simulink model "sm_stewart_platform"  (R2019a)
settings: Solver=ode45  StartTime=0.0  StopTime=40  MaxStep=0.001  RelTol=1e-3  EnableMultiTasking=on
model workspace (MAT data in the model file):
  g_density = 5
undefined symbols (not defined in the file or in its folder): B, nom_length, P, X, Y, Z
libraries: sm_lib x20, sm_stewart_platform_lib x8, nesl_utility x4
(part 1 of 3)
Description:
  | Stewart Platform
  | 
  | This model shows a Stewart platform manipulator that can track a
  | parameterized reference trajectory. The shape, size, and kinematics of
  | the manipulator are highly configurable.
  | 
  | The reference trajectory is
  | specified in 6-D pose space, and an inverse kinematics module
  | converts it into one through 6-D leg position space.  A generic PID
  | controller attempts to drive the manipulator along the desired
  | trajectory.
  | 
  | 
  | Copyright 2011-2018 The MathWorks, Inc.
settings Model: FPTRunName=Active  Creator=MathWorks  LastModifiedBy=Cybaster
settings DataIOCC: LimitDataPoints=on  SaveFormat=Array  SignalLoggingSaveFormat=ModelDataLogs  ReturnWorkspaceOutputs=off
settings OptimizationCC: ExpressionDepthLimit=2147483647  LifeSpan=inf
settings DebuggingCC: UnderspecifiedInitializationDetection=Classic  MergeDetectMultiDrivingBlocksExec=none  SolverPrmCheckMsg=warning  FcnCallInpInsideContextMsg=warning  StateNameClashWarn=warning  SFUnexpectedBacktrackingDiag=warning  SFNoUnconditionalDefaultTransitionDiag=warning  SFExecutionAtInitializationDiag=none  ArithmeticOperatorsInVariantConditions=warning
settings HardwareCC: ProdBitPerPointer=32  ProdBitPerSizeT=32  ProdBitPerPtrDiffT=32  ProdLargestAtomicFloat=None  ProdIntDivRoundTo=Undefined  ProdEndianess=Unspecified  ProdWordSize=32  ProdHWDeviceType=32-bit Generic
settings ModelReferenceCC: PropagateSignalLabelsOutOfModel=off
settings SFSimCC: SimUseLocalCustomCode=off
settings RTWCC: RTWUseLocalCustomCode=off
settings CodeAppCC: StateflowObjectComments=on
settings GRTTargetCC: TargetLangStandard=C89/C90 (ANSI)  GeneratePreprocessorConditionals=Disable all  CombineOutputUpdateFcns=off  GRTInterface=on
settings ConfigComp: CovMetricSettings=dw  CovHtmlReporting=on  CovSaveCumulativeToWorkspaceVar=on  CovSaveSingleToWorkspaceVar=on  CovExternalEMLEnable=off
settings SimscapeCC: SimscapeNormalizeSystem=off  SimscapeLogDataHistory=15000
settings ConfigurationSet: Description=SimMechanics 2G

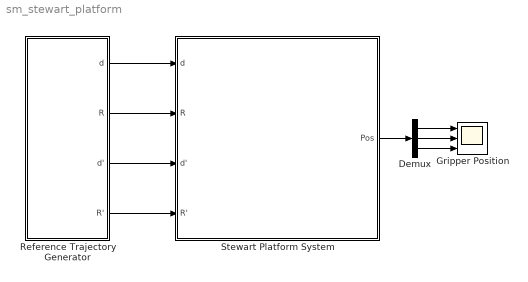
== system sm_stewart_platform ==
  Demux : Demux  Outputs=3
  Gripper Position : Scope  NumInputPorts=3
  Reference Trajectory Generator : Subsystem  mask(3-D Transform Trajectory Generator){Ax=0, wx=0, px=0, kx=0, Ay=0, wy=0, py=0, ky=0, Az=4, wz=180 / 10, pz=-90, kz=75, Aa=10, wa=360 * 3 / 10, pa=0, ka=0, Ab=10, wb=360 * 3 / 10, pb=-90, kb=0, Ac=0, wc=0, pc=0, kc=0}
      mask prompts: Ax "X Displacement Amplitude (cm)"; wx "X Displacement Frequency (deg / s)"; px "X Displacement Phase (deg)"; kx "X Displacement Offset (cm)"; Ay "Y Displacement Amplitude (cm)"; wy "Y Displacement Frequency (deg / s)"; py "Y Displacement Phase (deg)"; ky "Y Displacement Offset (cm)"; Az "Z Displacement Amplitude (cm)"; wz "Z Displacement Frequency (deg / s)"; pz "Z Displacement Phase (deg)"; kz "Z Displacement Offset (cm)"; Aa "X Rotation Amplitude (deg)"; wa "X Rotation Frequency (deg / s)"; pa "X Rotation Phase (deg)"; ka "X Rotation Offset (deg)"; Ab "Y Rotation Amplitude (deg)"; wb "Y Rotation Frequency (deg / s)"; pb "Y Rotation Phase (deg)"; kb "Y Rotation Offset (deg)"; Ac "Z Rotation Amplitude (deg)"; wc "Z Rotation Frequency (deg / s)"; pc "Z Rotation Phase (deg)"; kc "Z Rotation Offset (deg)"
      mask help: Tool for generating a wide variety of trajectories for a time-varying, 3-D rigid transformation between two frames.
      mask Help:
      | A <em>3-D Transform Trajectory Generator</em> is a tool for generating a wide variety of trajectories for a time-varying, 3-D rigid transformation between two frames.
      | 
      | A rigid transformation between two frames is characterized by a displacement vector and a rotation matrix.  Each of these can be parameterized with three scalar coordinates.  This block allows these six scalar coordinates to be parametrically specified as arbitrary sinusoidal functions of time.  The resulting displacement vector and rotation matrix, and their first derivatives are provided on the output ports.
      | 
      | <h3>Sinsoidal Functions</h3>
      | 
      | An arbitrary sinusoidal function of time is given by
      | 
      |     f(t) = A sin (w t + p) + k,
      | 
      | where <em>t</em> is time, and <em>A, w, p,</em> and <em>k</em> are scalar constants with the following meanings:
      | <ul>
      | <li> <em>A</em> is the <em>amplitude</em> of the sinusoid.
      | <li> <em>w</em> is the <em>angular frequency</em> of the sinusoid.
      | <li> <em>p</em> is the <em>phase</em> of the sinusoid.
      | <li> <em>k</em> is the <em>offset</em> of the sinusoid.
      | </ul>
      | 
      | <h3>Rigid Transformations</h3>
      | 
      | The time-varying, 3-D rigid transformation provided on the output ports of this block is, in turn, a function of scalar functions.  The displacement vector of the rigid transformation is given by:
      | 
      |     <b>d</b>(t) = [ x(t), y(t), z(t) ]^T
      | 
      | where x(t), y(t), and z(t) are scalar functions of time.
      | 
      | The rotation matrix of the rigid transformation is given by:
      | 
      |     <b>R</b>(t) = <b>R_x</b>(a(t)) <b>R_y</b>(b(t)) <b>R_z</b>(c(t)),
      | 
      | where a(t), b(t), and c(t) are scalar functions of time, and <b>R_x</b>, <b>R_y</b>, and <b>R_z</b> are rotations about the x, y, and z axes, respectively.
      | 
      | Note that this is an Euler angle parameterization of rotation.  The final rotation maps directions from a rotating frame F to a fixed frame G.  Beginning with F and G in an aligned configuration, the full rotation can be realized as a sequence of three rotations: first rotate F about its x-axis, then rotate F about its y-axis, and finally rotate F about its z-axis.  Alternatively, the rotation can be realized in a fixed-frame manner: first rotate F about G's z-axis, then rotate F about G's y-axis, and finally rotate F about G's z-axis. Both interpretations are correct.
      | 
      | The six scalar functions x(t), y(t), z(t), a(t), b(t), and c(t) are all arbitrary sinusoidal functions.  Each is parameterized by the four constants described in the preceding section.  This block computes these functions, and uses them to build the displacement vector, the rotation matrix, and the first time derivatives of these quantities.
      | 
      | 
      | <h3>Parameters</h3>
      | 
      | Each of the six parameter tabs defines four scalar parameters that together specify an arbitrary sinusoidal function of time, as described above.  The six tabs are:
      | 
      | <ul>
      | 
      | <li> <b>dx</b> Specifies the x-component of the displacement vector as a sinusoidal function of time.
      | 
      | <li> <b>dy</b> Specifies the y-component of the displacement vector as a sinusoidal function of time.
      | 
      | <li> <b>dz</b> Specifies the z-component of the displacement vector as a sinusoidal function of time.
      | 
      | <li> <b>Rx</b> Specifies the scalar rotation about the x-axis, part of the three-stage rotation sequence, as a sinusoidal function of time.
      | 
      | <li> <b>Ry</b> Specifies the scalar rotation about the y-axis, part of the three-stage rotation sequence, as a sinusoidal function of time.
      | 
      | <li> <b>Rz</b> Specifies the scalar rotation about the z-axis, part of the three-stage rotation sequence, as a sinusoidal function of time.
      | 
      | </ul>
      | 
      | <h3>Ports</h3>
      | 
      | <ul>
      | 
      | 
      | <li><b>d</b> The displacement vector of the time-varying, 3-D rigid transformation as a signal output.  This value is a 3 x 1 vector in units of centimeters.
      | 
      | <li><b>R</b> The rotation matrix of the time-varying, 3-D rigid transformation as a signal output.  This value is a 3 x 3 orthogonal matrix with +1 determinant.
      | 
      | <li><b>d'</b> The first time derivative of the signal appearing on the <em>d</em> port: a 3 x 1 vector in units of centimeters/second.
      | 
      | <li><b>R'</b> The first time derivative of the signal appearing on the <em>R</em> port: a 3 x 3 matrix.
      | 
      | </ul>
  Stewart Platform System : Subsystem  mask(Stewart Platform System){base_rad=28, base_thick=8, platform_rad=18, platform_thick=2, hex_skew=-0.25, upper_leg_len=10, lower_leg_len=14, leg_rad=3, collar_thick=0.5, gripper_height=30, claw_length=8, claw_width=3, claw_thick=1, end_eff_base_thick=2, flange_len=3, flange_width=2.25, flange_thick=.8, ic_R=eye(3), ic_d=[0 0 71]', Kp=300, Ki=20, Kd=5}
      mask prompts: base_rad "Base Radius  (cm)"; base_thick "Base Thickness (cm)"; platform_rad "Platform Radius (cm)"; platform_thick "Platform Thickness (cm)"; hex_skew "Hexagon Skew"; upper_leg_len "Upper Leg Length (cm)"; lower_leg_len "Lower Leg Length (cm)"; leg_rad "Leg Radius (cm)"; collar_thick "Collar Thickness (cm)"; gripper_height "Gripper Height (cm)"; claw_length "Claw Length (cm)"; claw_width "Claw Width (cm)"; claw_thick "Claw Thickness (cm)"; end_eff_base_thick "Base Thickness (cm)"; flange_len "Flange Length (cm)"; flange_width "Flange Width (cm)"; flange_thick "Flange Thickness (cm)"; ic_R "Rotation Matrix [3 x 3]"; ic_d "Displacement Vector (cm) [3 x 1]"; Kp "Controller Proportional Gain (N / cm)"; Ki "Controller Integral Gain (N / (cm s))"; Kd "Controller Derivative Gain (N / (cm / s)))"
      mask help:
      | Models a complete Stewart platform manipulator system.  The system can be driven to position and orient a special gripper frame according to specified trajectories.
      |
      | The system comprises a mechanical manipulator, an inverse kinematics module, and a control system.
      mask init:
      | params = struct( ...
      |     'base_thick',        base_thick,     ...
      |     'base_radius',       base_rad,       ...
      |     'platform_thick',    platform_thick, ...
      |     'platform_radius',   platform_rad,   ...
      |     'skew',              hex_skew,       ...
      |     'flange_length',     flange_len,     ...
      |     'flange_width',      flange_width,   ...
      |     'flange_thick',      flange_thick,   ...
      |     'leg_radius',        leg_rad,        ...
      |     'upper_leg_length',  upper_leg_len,  ...
      |     'lower_leg_length',  lower_leg_len,  ...
      |     'gripper_height',    gripper_height  ...
      |     );
      | 
      | [B, P, nom_length] = sm_stewart_platform_setup(params);
      | 
      | lengths = sm_stewart_platform_ik(B, P, nom_length, ic_R, ic_d);
      mask Help:
      | A <em>Stewart Platform System</em> models a complete Stewart platform manipulator system.  The system can be driven to position and orient a special gripper frame according to specified trajectories.
      | 
      | <h3>Subsystems</h3>
      | 
      | A Stewart platform system comprises three primary subsystems:
      | 
      | <ol>
      | 
      | <li><b>Manipulator</b> The manipulator is the Simscape Multibody subsystem describing the mechanical structure of the Stewart platform.  The manipulator contains two hexagonal plates, a lower base plate and an upper platform plate, connected by six articulated legs.  The base plate is anchored to the world frame, and the platform plate is controlled to position and orient the gripper frame. The manipulator component provides sensing and actuation signals to interface to a controller.
      | 
      |   The manipulator is highly parameterized.  Most parameters of the Stewart platform system are physical lengths and other parameters that control the shapes and sizes of the components of the manipulator. By varying these parameters, a wide range of Stewart platform manipulators can be realized.
      | 
      | <li><b>Inverse Kinematics (IK) Module</b> The inverse kinematics module is a pure Simulink subsystem that maps time-varying signals describing the desired position and orientation of the gripper frame into time-varying scalar signals specifying the positions and velocities of the prismatic primitives of the leg joints.  This is an essential component of a complete Stewart platform system because the user of the system typically expresses a desired trajectory in the 6-D space of positions and orientations of the gripper frame, but the manipulator control is simplest in the 6-D space of leg joint positions. The IK module forms the bridge between these two spaces.
      | 
      |   The mathematics performed within the IK module is heavily dependent on the physical parameters that determine the shape and size of the manipulator itself.  Most of the parameters that govern the manipulator are also used within the IK module.
      | 
      | <li><b>Control System</b> The control system is a pure Simulink subsystem that attempts to drive the gripper frame along its desired trajectory by controlling the positions of the prismatic primitives of the leg joints. It uses a standard PID control scheme, with gains specified by Stewart platform system parameters.  The control uses no information about the forward or inverse kinematics of the platform; it simply tries to drive a point along a trajectory in 6-D space.
      | 
      |   The controller takes both the desired and actual leg position vectors and the first derivatives of these quantities.  It generates a 6-D commanded force output that can be used to drive the six leg lengths to thei desired values.
      | 
      |   Because the size and shape of the Stewart platform manipulator can vary significantly depending on the parameter settings, the controller gains may need to be adjusted in order to control the manipulator to the desired trajectory.
      | 
      | </ol>
      | 
      | <h3>Base and Platform Plates</h3>
      | 
      | The <em>Plates</em> tab parameters specify the geometry of the base and platform hexagon plates of the Stewart platform manipulator.  See the documentation of the <em>Hexagon Plate</em> library block for details.
      | 
      | <ul>
      | 
      | <li> <b>Base Radius</b> The radius of the base plate.  The vertices of the hexagonal cross section all lie on a circle of this radius.
      | 
      | <li> <b>Base Thickness</b> The thickness of the base plate.
      | 
      | <li> <b>Platform Radius</b> The radius of the platform plate.  The vertices of the hexagonal cross section all lie on a circle of this radius.
      | 
      | <li> <b>Platform Thickness</b> The thickness of the platform plate.
      | 
      | <li> <b>Hexagon Skew</b> The common skew factor of the base and platform plates. This value, in the range (-0.5, +0.5), determines the shape of the three-fold symmetric hexagons.  A zero skew factor produces regular hexagons.  As the skew factor magnitude increases, the hexagons become more triangular.
      | 
      | </ul>
      | 
      | <h3>Legs</h3>
      | 
      | The <em>Legs</em> tab parameters specify the common geometry of the six legs of the Stewart platform manipulator.  See the documentation of the <em>Leg</em> library block for details.
      | 
      | <ul>
      | 
      | <li> <b>Upper Leg Length</b> The length of the upper leg, including its end collars.
      | 
      | <li> <b>Lower Leg Length</b> The length of the lower leg, including its end collars.
      | 
      | <li> <b>Leg Radius</b> The common radius of the upper and lower leg segments. Each segment's cross section is a regular hexagon inscribed in a circle of this radius.
      | 
      | <li> <b>Collar Thickness</b> The thickness of the hexagonal collars adjoined to the ends of each leg segment.
      | 
      | </ul>
      | 
      | <h3>End Effector</h3>
      | 
      | The <em>End Eff</em> tab parameters specify the geometry of the end effector attached to the platform plate of the Stewart platform manipulator. See the documentation of the <em>End Effector</em> block within the <em>Manipulator</em> subsystem for details.
      | 
      | <ul>
      | 
      | <li> <b>Gripper Height</b> The vertical distance from the origin of the gripper frame to the top surface of the movable platform plate.
      | 
      | <li> <b>Claw Length</b> The length (height) of the trapezoidal claws of the gripper.
      | 
      | <li> <b>Claw Width</b> The width of the trapezoidal claws of the gripper where they attach to the gripper base.
      | 
      | <li> <b>Claw Thickness</b> The thickness of the trapezoidal claws of the gripper.
      | 
      | <li> <b>Base Thickness</b> The thickness of the triangular gripper base.
      | 
      | </ul>
      | 
      | <h3>Flanges</h3>
      | 
      | The <em>Flanges</em> tab parameters specify the common geometry of the 48 flanges attached to the hexagonal plates and legs of the Stewart platform manipulator.  Each of the 12 universal joints is supported by four flanges.  See the documentation of the <em>Flange</em> library block for details.
      | 
      | <ul>
      | 
      | <li> <b>Flange Length</b> The length of the rectangular prism portion of the flanges.
      | 
      | <li> <b>Flange Width</b> The width of the rectangular prism portion of the flanges.
      | 
      | <li> <b>Flange Thickness</b> The thickness of the flanges.
      | 
      | </ul>
      | 
      | <h3>Initial Conditions</h3>
      | 
      | The <em>IC</em> tab parameters specify the initial conditions of the Stewart Platform manipulator for simulation.  Specifically, these specify the <em>position</em> of the manipulator; the simulation always starts from a rest (zero velocity) state.
      | 
      | The initial position is defined by specifying pose of the gripper frame relative to the world frame.  This is typically a convenient parameterization for a user of the manipulator.  The world frame is also the reference frame of the manipulator base plate.  This is a frame with origin at the center of the manipulator base (which is in its interior), and with z-axis pointed directly upward.
      | 
      | An Update Diagram (Ctrl-D) operation will attempt to assemble the manipulator in the specified initial position.  Some initial positions may be incompatible with the kinematics of the manipulator, based on other parameter settings.  In such cases, the assembly will fail.
      | 
      | Also note that if the initial position differs significantly from the desired trajectory (specified through the input signal ports) at time zero, the manipulator's motion may be subject to large transients at the start of simulation.
      | 
      | <ul>
      | 
      | <li> <b>Rotation Matrix</b> The rotation matrix mapping directions in the gripper frame to directions in the world frame.  This should be a 3 x 3 orthogonal matrix determinant +1.  The columns of this matrix are the canonical i, j, and k unit vectors of the gripper frame resolved in world frame coordinates.
      | 
      | <li> <b>Displacement Vector</b> The location of the origin of the gripper frame in world frame coordinates.  This should be a 3 x 1 column vector.  The z-coordinate should generally be positive, on the order of the nominal lengths of the legs.
      | 
      | </ul>
      | 
      | If the rotation matrix is the identity and the x- and y-coordinates of the displacement vector are zero, the initial configuration of the manipulator will be symmetric with all leg positions equal.
      | 
      | <h3>Controller Gains</h3>
      | 
      | The <em>Control</em> tab parameters specify the gains of the internal controller used to control the manipulator's pose according to a specified trajectory.  The controller uses a generic PID control scheme.  The gains may need to be adjusted to be appropriate if the parameters governing the size and kinematics of the manipulator are changed significantly.
      | 
      | See the documentation of the <em>Controller</em> subsystem for details.
      | 
      | <ul>
      | 
      | <li> <b>Controller Proportional Gain</b> The proportional (P) gain of the internal PID controller.
      | 
      | <li> <b>Controller Integral Gain</b> The integral (I) gain of the internal PID controller.
      | 
      | <li> <b>Controller Derivative Gain</b> The derivative (D) gain of the internal PID controller.
      | 
      | </ul>
      | 
      | 
      | 
      | <h3>Ports</h3>
      | 
      | <ul>
      | 
      | <li><b>d</b> The desired displacement vector of the gripper frame relative to the world frame as a signal input.  This value should be a 3 x 1 vector in units of centimeters.  It specifies the desired origin of the gripper frame in world frame coordinates as a function of time.  This signal is analogous to the <em>Displacement Vector</em> on the <em>IC</em> parameter tab.
      | 
      | <li><b>R</b> The desired rotation matrix from the gripper frame to the world frame as a signal input.  This value should be a 3 x 3 orthogonal matrix with +1 determinant.  The columns of this matrix are the canonical i, j, and k unit vectors of the gripper frame resolved in world frame coordinates, specified as functions of time.  This signal is analogous to the <em>Rotation Matrix</em> on the <em>IC</em> parameter tab.
      | 
      | <li><b>d'</b> The first time derivative of the desired displacement vector of the gripper frame relative to the world frame as a signal input.  This value should be the first time derivative of the signal provided on the <em>d</em> port: a 3 x 1 vector in units of centimeters/second. It specifies the velocity of the origin of the gripper frame in  world frame coordinates as a function of time.
      | 
      | <li><b>R'</b> The first time derivative of the desired rotation matrix from the gripper frame to the world frame as a signal input.  This value should be the first time derivative of the signal provided on the <em>R</em> port: a 3 x 3 matrix.
      | 
      | <li><b>Pos</b> The position of the gripper with respect to the world frame as a 3 x 1 position vector in units of centimeters.
      | </ul>
      | 
      | <!--  LocalWords:  Eff IC Ctrl IK
      |  -->
      mask Display:
      | image(imread('sm_stewart_platform_system.png'))
      | color('yellow')
      | port_label('Input', 1, 'd')
      | port_label('Input', 2, 'R')
      | port_label('Input', 3, 'd''')
      | port_label('Input', 4, 'R''')
      | port_label('Output', 1, 'Pos')
  wires:
  Reference Trajectory Generator/1(d) -> Stewart Platform System/1(d)
  Reference Trajectory Generator/2(R) -> Stewart Platform System/2(R)
  Reference Trajectory Generator/3(d') -> Stewart Platform System/3(d')
  Reference Trajectory Generator/4(R') -> Stewart Platform System/4(R')
  Stewart Platform System/1(Pos) -> Demux/1
  Demux/1 -> Gripper Position/1
  Demux/2 -> Gripper Position/2
  Demux/3 -> Gripper Position/3

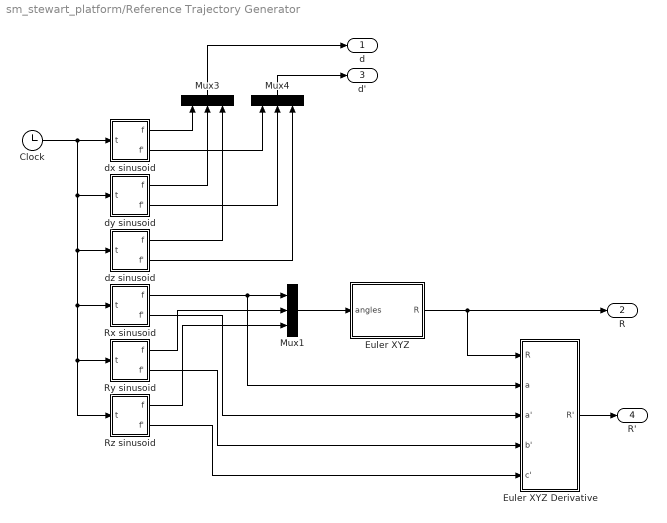
== system sm_stewart_platform/Reference Trajectory Generator ==
  Clock : Clock
  Euler XYZ : Subsystem  mask(Euler XYZ){}
      mask help: Converts a set of Euler angles to the corresponding rotation matrix from rotated frame to fixed frame coordinates.
      mask Help:
      | An <em>Euler XYZ</em>  block converts a set of Euler angles to the corresponding
      |   rotation matrix from rotated frame to fixed frame coordinates.
      | 
      | Arbitrary 3-D rotations can be parameterized by a vector of three Euler angles:
      |   a, b, and c.  The resulting rotation is given by
      | 
      |     <b>R</b> = <b>R_x</b>(a) <b>R_y</b>(b) <b>R_z</b>(c).
      | 
      | where <b>R_x</b>, <b>R_y</b>, and <b>R_z</b> are rotations about the x, y, and z
      | axes, respectively.
      | 
      | The complete rotation <b>R</b> maps directions from a rotated frame F to a
      | fixed frame G.  Beginning with F and G in an aligned configuration, the full
      | rotation can be realized as a sequence of three rotations: first rotate F
      | about its x-axis, then rotate F about its y-axis, and finally rotate F about its
      | z-axis.  Alternatively, the rotation can be realized in a fixed-frame manner:
      | first rotate F about G's z-axis, then rotate F about G's y-axis, and finally
      | rotate F about G's z-axis.  Both interpretations are correct.
      | 
      | 
      | <h3>Ports</h3>
      | 
      | <ul>
      | 
      | <li> <b>angles</b> The Euler angles a, b, and c (in that order) as a 3-vector
      |   with units of radians.
      | 
      | <li> <b>R</b> The resulting rotation matrix.  This matrix is always a 3 x 3
      | orthogonal matrix with a +1 determinant.
      | 
      | </ul>
  Euler XYZ Derivative : Subsystem  mask(Euler XYZ Derivative){}
      mask help: Computes the first time derivative of a rotation matrix specified by a set of Euler angles.
      mask Help:
      | An <em>Euler XYZ Derivative</em>  block computes the first time derivative of a
      |  rotation matrix specified by a set of Euler angles.
      | 
      | Arbitrary 3-D rotations can be parameterized by a vector of three Euler angles:
      |   a, b, and c.  The resulting rotation is given by
      | 
      |     <b>R</b> = <b>R_x</b>(a) <b>R_y</b>(b) <b>R_z</b>(c).
      | 
      | where <b>R_x</b>, <b>R_y</b>, and <b>R_z</b> are rotations about the x, y, and z
      | axes, respectively.
      | 
      | If a, b, and c are, in turn, functions of time, with instantaneous derivatives
      | a', b', and c', then <b>R'</b>, the time derivative of <b>R</b> is given by
      | 
      |     <b>R'</b> = a' <b>i~ R_x</b>(a) <b>R_y</b>(b) <b>R_z</b>(c) + b' <b>R_x</b>(a) <b>j~ R_y</b>(b) <b>R_z</b>(c) + c' <b>R_x</b>(a) <b>R_y</b>(b) <b>k~ R_z</b>(c),
      | 
      | where <b>~</b> is the canonical operator converting a 3-vector <b>v</b> into a
      | corresponding 3 x 3 skew-symmetric matrix <b>v~</b> such that
      | 
      |     <b>v~ u</b> = <b>v</b> x <b>u</b> for all <b>u</b>.
      | 
      | With some vector algebra, the above expression of <b>R'</b> can be simplified to
      | 
      |     <b>R'</b> = [a' <b>i</b> + b' <b>R_x</b>(a) <b>j</b> ]<b>~</b> <b>R</b> + c' <b>[+R_2, -R_1, 0]</b>
      | 
      | where <b>R_i</b> is the ith column of <b>R</b>.
      | 
      | The block computes the value of <b>R'</b> according to the last equation above.
      | In addition to <b>R</b>, the computation requires the scalar Euler
      | angle <em>a</em>, and the time derivatives of all three Euler angles.
      | 
      | 
      | <h3>Ports</h3>
      | 
      | <ul>
      | 
      | <li> <b>R</b> The rotation matrix defined by the Euler angles <em>a, b,</em>
      | and <em>c</em> (see above).
      | 
      | <li> <b>a</b> The Euler angle corresponding to rotation about the x-axis.
      | 
      | <li> <b>a'</b> The time derivative of the Euler angle corresponding to rotation
      | about the x-axis.
      | 
      | <li> <b>b'</b> The time derivative of the Euler angle corresponding to rotation
      | about the y-axis.
      | 
      | <li> <b>c'</b> The time derivative of the Euler angle corresponding to rotation
      | about the z-axis.
      | 
      | </ul>
  Mux1 : Mux  Inputs=3
  Mux3 : Mux  Inputs=3
  Mux4 : Mux  Inputs=3
  Rx sinusoid : Subsystem  mask(Sinusoidal Trajectory){A=Aa * pi/180, w=wa, p=pa, k=ka * pi/180}
      mask prompts: A "Amplitude"; w "Frequency (deg / s)"; p "Phase (deg)"; k "Offset"
      mask help: Produces a time-varying sinusoid parameterized by amplitude, frequency, phase, and offset. Also produces the first time derivative of this function.
      mask Help:
      | A <em>Sinusoidal Trajectory</em> produces a time-varying sinusoid
      |  parameterized by amplitude, frequency, phase, and offset.  It also produces the
      |  first time derivative of this function.
      | 
      | <h3>Sinsoidal Functions</h3>
      | 
      | An arbitrary sinusoidal function of time and its first time derivative are given by
      | 
      |     f(t) = A sin (w t + p) + k
      |     f'(t) = w A cos (w t + p),
      | 
      | where <em>t</em> is time, and <em>A, w, p,</em> and <em>k</em> are scalar
      | constants.  Given time as an input signal, this block provides the f(t) and
      | f'(t) signals based on the parameters described above.
      | 
      | 
      | <h3>Parameters</h3>
      | 
      | The four parameters specify the scalar parameters described above:
      | 
      | <ul>
      | 
      | <li> <b>A</b> The <em>amplitude</em> of the sinusoid.
      | 
      | <li> <b>w</b> The <em>angular frequency</em> of the sinusoid.
      | 
      | <li> <b>p</b> The <em>phase</em> of the sinusoid.
      | 
      | <li> <b>k</b> The <em>offset</em> of the sinusoid.
      | 
      | </ul>
      | 
      | </ul>
      | 
      | <h3>Ports</h3>
      | 
      | <ul>
      | 
      | <li><b>t</b> The time function, provided as an input signal.
      | 
      | <li><b>f</b> The sinusoid f(t), as described above, as an output signal.
      | 
      | <li><b>f'</b> The sinusoid's first time derivative f'(t), as described above, as an output signal.
      | 
      | </ul>
  Ry sinusoid : Subsystem  mask(Sinusoidal Trajectory){A=Ab * pi/180, w=wb, p=pb, k=kb * pi/180}
      mask prompts: A "Amplitude"; w "Frequency (deg / s)"; p "Phase (deg)"; k "Offset"
      mask help: Produces a time-varying sinusoid parameterized by amplitude, frequency, phase, and offset. Also produces the first time derivative of this function.
      mask Help:
      | A <em>Sinusoidal Trajectory</em> produces a time-varying sinusoid
      |  parameterized by amplitude, frequency, phase, and offset.  It also produces the
      |  first time derivative of this function.
      | 
      | <h3>Sinsoidal Functions</h3>
      | 
      | An arbitrary sinusoidal function of time and its first time derivative are given by
      | 
      |     f(t) = A sin (w t + p) + k
      |     f'(t) = w A cos (w t + p),
      | 
      | where <em>t</em> is time, and <em>A, w, p,</em> and <em>k</em> are scalar
      | constants.  Given time as an input signal, this block provides the f(t) and
      | f'(t) signals based on the parameters described above.
      | 
      | 
      | <h3>Parameters</h3>
      | 
      | The four parameters specify the scalar parameters described above:
      | 
      | <ul>
      | 
      | <li> <b>A</b> The <em>amplitude</em> of the sinusoid.
      | 
      | <li> <b>w</b> The <em>angular frequency</em> of the sinusoid.
      | 
      | <li> <b>p</b> The <em>phase</em> of the sinusoid.
      | 
      | <li> <b>k</b> The <em>offset</em> of the sinusoid.
      | 
      | </ul>
      | 
      | </ul>
      | 
      | <h3>Ports</h3>
      | 
      | <ul>
      | 
      | <li><b>t</b> The time function, provided as an input signal.
      | 
      | <li><b>f</b> The sinusoid f(t), as described above, as an output signal.
      | 
      | <li><b>f'</b> The sinusoid's first time derivative f'(t), as described above, as an output signal.
      | 
      | </ul>
  Rz sinusoid : Subsystem  mask(Sinusoidal Trajectory){A=Ac * pi/180, w=wc, p=pc, k=kc * pi/180}
      mask prompts: A "Amplitude"; w "Frequency (deg / s)"; p "Phase (deg)"; k "Offset"
      mask help: Produces a time-varying sinusoid parameterized by amplitude, frequency, phase, and offset. Also produces the first time derivative of this function.
      mask Help:
      | A <em>Sinusoidal Trajectory</em> produces a time-varying sinusoid
      |  parameterized by amplitude, frequency, phase, and offset.  It also produces the
      |  first time derivative of this function.
      | 
      | <h3>Sinsoidal Functions</h3>
      | 
      | An arbitrary sinusoidal function of time and its first time derivative are given by
      | 
      |     f(t) = A sin (w t + p) + k
      |     f'(t) = w A cos (w t + p),
      | 
      | where <em>t</em> is time, and <em>A, w, p,</em> and <em>k</em> are scalar
      | constants.  Given time as an input signal, this block provides the f(t) and
      | f'(t) signals based on the parameters described above.
      | 
      | 
      | <h3>Parameters</h3>
      | 
      | The four parameters specify the scalar parameters described above:
      | 
      | <ul>
      | 
      | <li> <b>A</b> The <em>amplitude</em> of the sinusoid.
      | 
      | <li> <b>w</b> The <em>angular frequency</em> of the sinusoid.
      | 
      | <li> <b>p</b> The <em>phase</em> of the sinusoid.
      | 
      | <li> <b>k</b> The <em>offset</em> of the sinusoid.
      | 
      | </ul>
      | 
      | </ul>
      | 
      | <h3>Ports</h3>
      | 
      | <ul>
      | 
      | <li><b>t</b> The time function, provided as an input signal.
      | 
      | <li><b>f</b> The sinusoid f(t), as described above, as an output signal.
      | 
      | <li><b>f'</b> The sinusoid's first time derivative f'(t), as described above, as an output signal.
      | 
      | </ul>
  dx sinusoid : Subsystem  mask(Sinusoidal Trajectory){A=Ax, w=wx, p=px, k=kx}
      mask prompts: A "Amplitude"; w "Frequency (deg / s)"; p "Phase (deg)"; k "Offset"
      mask help: Produces a time-varying sinusoid parameterized by amplitude, frequency, phase, and offset. Also produces the first time derivative of this function.
      mask Help:
      | A <em>Sinusoidal Trajectory</em> produces a time-varying sinusoid
      |  parameterized by amplitude, frequency, phase, and offset.  It also produces the
      |  first time derivative of this function.
      | 
      | <h3>Sinsoidal Functions</h3>
      | 
      | An arbitrary sinusoidal function of time and its first time derivative are given by
      | 
      |     f(t) = A sin (w t + p) + k
      |     f'(t) = w A cos (w t + p),
      | 
      | where <em>t</em> is time, and <em>A, w, p,</em> and <em>k</em> are scalar
      | constants.  Given time as an input signal, this block provides the f(t) and
      | f'(t) signals based on the parameters described above.
      | 
      | 
      | <h3>Parameters</h3>
      | 
      | The four parameters specify the scalar parameters described above:
      | 
      | <ul>
      | 
      | <li> <b>A</b> The <em>amplitude</em> of the sinusoid.
      | 
      | <li> <b>w</b> The <em>angular frequency</em> of the sinusoid.
      | 
      | <li> <b>p</b> The <em>phase</em> of the sinusoid.
      | 
      | <li> <b>k</b> The <em>offset</em> of the sinusoid.
      | 
      | </ul>
      | 
      | </ul>
      | 
      | <h3>Ports</h3>
      | 
      | <ul>
      | 
      | <li><b>t</b> The time function, provided as an input signal.
      | 
      | <li><b>f</b> The sinusoid f(t), as described above, as an output signal.
      | 
      | <li><b>f'</b> The sinusoid's first time derivative f'(t), as described above, as an output signal.
      | 
      | </ul>
  dy sinusoid : Subsystem  mask(Sinusoidal Trajectory){A=Ay, w=wy, p=py, k=ky}
      mask prompts: A "Amplitude"; w "Frequency (deg / s)"; p "Phase (deg)"; k "Offset"
      mask help: Produces a time-varying sinusoid parameterized by amplitude, frequency, phase, and offset. Also produces the first time derivative of this function.
      mask Help:
      | A <em>Sinusoidal Trajectory</em> produces a time-varying sinusoid
      |  parameterized by amplitude, frequency, phase, and offset.  It also produces the
      |  first time derivative of this function.
      | 
      | <h3>Sinsoidal Functions</h3>
      | 
      | An arbitrary sinusoidal function of time and its first time derivative are given by
      | 
      |     f(t) = A sin (w t + p) + k
      |     f'(t) = w A cos (w t + p),
      | 
      | where <em>t</em> is time, and <em>A, w, p,</em> and <em>k</em> are scalar
      | constants.  Given time as an input signal, this block provides the f(t) and
      | f'(t) signals based on the parameters described above.
      | 
      | 
      | <h3>Parameters</h3>
      | 
      | The four parameters specify the scalar parameters described above:
      | 
      | <ul>
      | 
      | <li> <b>A</b> The <em>amplitude</em> of the sinusoid.
      | 
      | <li> <b>w</b> The <em>angular frequency</em> of the sinusoid.
      | 
      | <li> <b>p</b> The <em>phase</em> of the sinusoid.
      | 
      | <li> <b>k</b> The <em>offset</em> of the sinusoid.
      | 
      | </ul>
      | 
      | </ul>
      | 
      | <h3>Ports</h3>
      | 
      | <ul>
      | 
      | <li><b>t</b> The time function, provided as an input signal.
      | 
      | <li><b>f</b> The sinusoid f(t), as described above, as an output signal.
      | 
      | <li><b>f'</b> The sinusoid's first time derivative f'(t), as described above, as an output signal.
      | 
      | </ul>
  dz sinusoid : Subsystem  mask(Sinusoidal Trajectory){A=Az, w=wz, p=pz, k=kz}
      mask prompts: A "Amplitude"; w "Frequency (deg / s)"; p "Phase (deg)"; k "Offset"
      mask help: Produces a time-varying sinusoid parameterized by amplitude, frequency, phase, and offset. Also produces the first time derivative of this function.
      mask Help:
      | A <em>Sinusoidal Trajectory</em> produces a time-varying sinusoid
      |  parameterized by amplitude, frequency, phase, and offset.  It also produces the
      |  first time derivative of this function.
      | 
      | <h3>Sinsoidal Functions</h3>
      | 
      | An arbitrary sinusoidal function of time and its first time derivative are given by
      | 
      |     f(t) = A sin (w t + p) + k
      |     f'(t) = w A cos (w t + p),
      | 
      | where <em>t</em> is time, and <em>A, w, p,</em> and <em>k</em> are scalar
      | constants.  Given time as an input signal, this block provides the f(t) and
      | f'(t) signals based on the parameters described above.
      | 
      | 
      | <h3>Parameters</h3>
      | 
      | The four parameters specify the scalar parameters described above:
      | 
      | <ul>
      | 
      | <li> <b>A</b> The <em>amplitude</em> of the sinusoid.
      | 
      | <li> <b>w</b> The <em>angular frequency</em> of the sinusoid.
      | 
      | <li> <b>p</b> The <em>phase</em> of the sinusoid.
      | 
      | <li> <b>k</b> The <em>offset</em> of the sinusoid.
      | 
      | </ul>
      | 
      | </ul>
      | 
      | <h3>Ports</h3>
      | 
      | <ul>
      | 
      | <li><b>t</b> The time function, provided as an input signal.
      | 
      | <li><b>f</b> The sinusoid f(t), as described above, as an output signal.
      | 
      | <li><b>f'</b> The sinusoid's first time derivative f'(t), as described above, as an output signal.
      | 
      | </ul>
  d : Outport
  R : Outport  Port=2
  d' : Outport  Port=3
  R' : Outport  Port=4
  wires:
  dx sinusoid/1(f) -> Mux3/1
  dy sinusoid/1(f) -> Mux3/2
  dz sinusoid/1(f) -> Mux3/3
  dx sinusoid/2(f') -> Mux4/1
  dy sinusoid/2(f') -> Mux4/2
  dz sinusoid/2(f') -> Mux4/3
  Mux3/1 -> d/1
  Mux4/1 -> d'/1
  Rx sinusoid/1(f) -> Mux1/1, Euler XYZ Derivative/2(a)
  Euler XYZ Derivative/1(R') -> R'/1
  Clock/1 -> Ry sinusoid/1(t), Rz sinusoid/1(t), Rx sinusoid/1(t), dz sinusoid/1(t), dy sinusoid/1(t), dx sinusoid/1(t)
  Ry sinusoid/1(f) -> Mux1/2
  Rz sinusoid/1(f) -> Mux1/3
  Rx sinusoid/2(f') -> Euler XYZ Derivative/3(a')
  Ry sinusoid/2(f') -> Euler XYZ Derivative/4(b')
  Rz sinusoid/2(f') -> Euler XYZ Derivative/5(c')
  Mux1/1 -> Euler XYZ/1(angles)
  Euler XYZ/1(R) -> R/1, Euler XYZ Derivative/1(R)
